simulink model "Simple_LQR"  (R2020b)
settings: Solver=VariableStepAuto  StartTime=0.0  StopTime=10  FixedStep=TS  RelTol=1e-3
values from neighbouring files (symbols this model uses):
  k_f = K_lqr(1:4)    [SYSTEM_BALLBOT.m]
  k_i = K_lqr(5)    [SYSTEM_BALLBOT.m]
  XIV = [ ... (first row only)    [SYSTEM_BALLBOT.m]
undefined symbols (not defined in the file or in its folder): A, B, C, D, Kb, Kp, Ra, Rs, Rw
settings Model: Creator=ADMIN  LastModifiedBy=ADMIN
settings DataIOCC: SaveFormat=Array  SaveOutput=off  SignalLogging=off  DSMLogging=off  ReturnWorkspaceOutputs=off
settings DebuggingCC: UnconnectedInputMsg=none  UnconnectedOutputMsg=none  UnconnectedLineMsg=none
settings ModelReferenceCC: EnableRefExpFcnMdlSchedulingChecks=off
settings RTWCC: GPUComputeCapability=5.0
settings ConfigComp: CovBoundaryAbsTol=1.0e-5

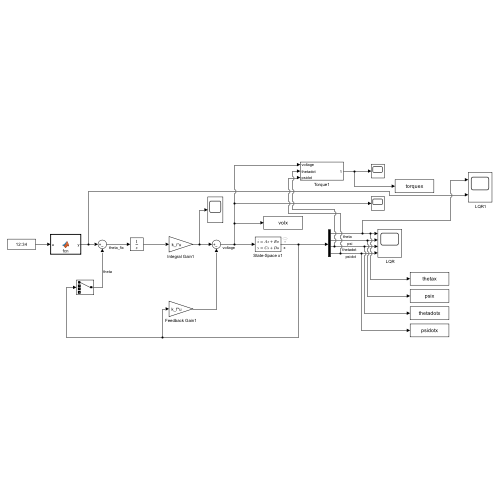
[thumbnail: Simulink's stored preview of the top-level diagram]
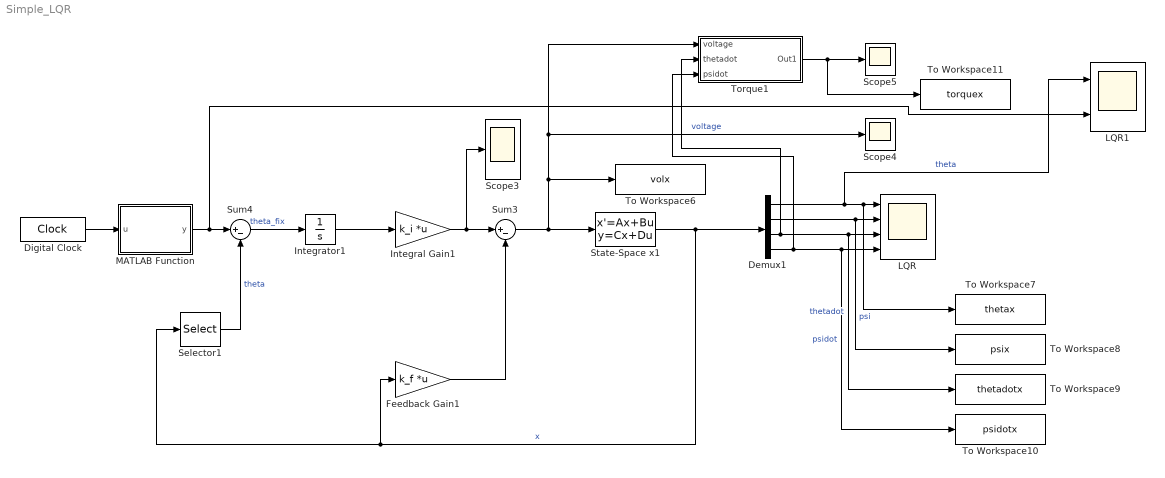
== system Simple_LQR ==
  " LQR" : Scope  NumInputPorts=4
  " LQR1" : Scope  NumInputPorts=2
  Demux1 : Demux
  Digital Clock : DigitalClock
  Feedback Gain1 : Gain  Gain=k_f  Multiplication=Matrix(K*u)  OutDataTypeStr=Inherit: Same as input  ParamDataTypeStr=Inherit: Same as input
  Integral Gain1 : Gain  Gain=k_i  Multiplication=Matrix(K*u)  OutDataTypeStr=Inherit: Same as input  ParamDataTypeStr=Inherit: Same as input
  Integrator1 : Integrator
  MATLAB Function : MATLAB Function  TreatAsAtomicUnit=on
  Scope3 : Scope
  Scope4 : Scope
  Scope5 : Scope
  Selector1 : Selector  InputPortWidth=4  IndexOptions=Index vector (dialog)  Indices=1  OutputSizes=1
  State-Space x1 : StateSpace  A=A  B=B  C=C  D=D  InitialCondition=XIV
  Sum3 : Sum  Inputs=|+-  OutDataTypeStr=Inherit: Same as first input
  Sum4 : Sum  Inputs=|+-  OutDataTypeStr=Inherit: Same as first input
  To Workspace10 : ToWorkspace  VariableName=psidotx  SampleTime=-1
      settings: Save2DSignal=2-D array (concatenate along first dimension)
  To Workspace11 : ToWorkspace  VariableName=torquex  SampleTime=-1
      settings: Save2DSignal=2-D array (concatenate along first dimension)
  To Workspace6 : ToWorkspace  VariableName=volx  SampleTime=-1
      settings: Save2DSignal=2-D array (concatenate along first dimension)
  To Workspace7 : ToWorkspace  VariableName=thetax  SampleTime=-1
      settings: Save2DSignal=2-D array (concatenate along first dimension)
  To Workspace8 : ToWorkspace  VariableName=psix  SampleTime=-1
      settings: Save2DSignal=2-D array (concatenate along first dimension)
  To Workspace9 : ToWorkspace  VariableName=thetadotx  SampleTime=-1
      settings: Save2DSignal=2-D array (concatenate along first dimension)
  Torque1 : Subsystem
  wires:
  Torque1/1(Out1) -> To Workspace11/1, Scope5/1
  Integrator1/1 -> Integral Gain1/1
  Demux1/4 -> Torque1/3(psidot), To Workspace10/1, " LQR"/4  "psidot"
  MATLAB Function/1(y) -> " LQR1"/2, Sum4/1
  State-Space x1/1 -> Selector1/1, Feedback Gain1/1, Demux1/1  "x"
  Demux1/3 -> Torque1/2(thetadot), To Workspace9/1, " LQR"/3  "thetadot"
  Demux1/2 -> To Workspace8/1, " LQR"/2  "psi"
  Feedback Gain1/1 -> Sum3/2
  Demux1/1 -> " LQR1"/1, To Workspace7/1, " LQR"/1  "theta"
  Selector1/1 -> Sum4/2  "theta"
  Sum3/1 -> State-Space x1/1, To Workspace6/1, Torque1/1(voltage), Scope4/1  "voltage"
  Integral Gain1/1 -> Scope3/1, Sum3/1
  Sum4/1 -> Integrator1/1  "theta_fix"
  Digital Clock/1 -> MATLAB Function/1(u)

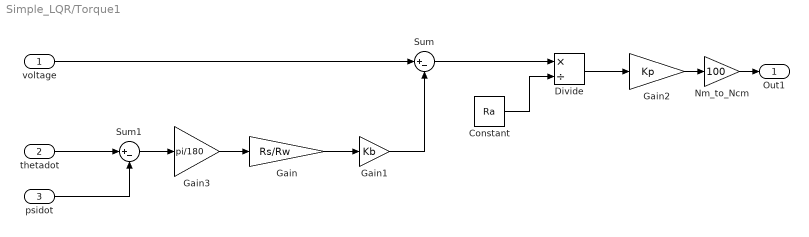
== system Simple_LQR/Torque1 ==
  voltage : Inport
  thetadot : Inport  Port=2
  psidot : Inport  Port=3
  Constant : Constant  Value=Ra
  Divide : Product  Inputs=*/
  Gain : Gain  Gain=Rs/Rw
  Gain1 : Gain  Gain=Kb
  Gain2 : Gain  Gain=Kp
  Gain3 : Gain  Gain=pi/180
  Nm_to_Ncm : Gain  Gain=100
  Sum : Sum  Inputs=|+-
  Sum1 : Sum  Inputs=|+-
  Out1 : Outport
  wires:
  voltage/1 -> Sum/1
  thetadot/1 -> Sum1/1
  psidot/1 -> Sum1/2
  Gain1/1 -> Sum/2
  Sum/1 -> Divide/1
  Constant/1 -> Divide/2
  Divide/1 -> Gain2/1
  Gain/1 -> Gain1/1
  Sum1/1 -> Gain3/1
  Gain3/1 -> Gain/1
  Gain2/1 -> Nm_to_Ncm/1
  Nm_to_Ncm/1 -> Out1/1

== matlab function Simple_LQR/MATLAB Function ==
  data: u input; y output
function y = fcn(u)
    if(u >= 0 && u <= 10)
        y = 0;
    else 
        y=100;
    end
